simulink model "audioThru"  (R2020b)
settings: Solver=FixedStepDiscrete  StartTime=0.0  StopTime=10.0  RelTol=1e-3
settings Model: DataTypeOverride=Off  Creator=amatsumo  LastModifiedBy=amatsumo
settings DataIOCC: SaveOutput=off  SaveTime=off
settings OptimizationCC: BlockReduction=off  ConditionallyExecuteInputs=off  DefaultParameterBehavior=Inlined
settings DebuggingCC: AlgebraicLoopMsg=error  SingleTaskRateTransMsg=error  StrictBusMsg=ErrorOnBusTreatedAsVector  ArithmeticOperatorsInVariantConditions=warning
settings HardwareCC: ProdBitPerPointer=32  ProdBitPerSizeT=32  ProdBitPerPtrDiffT=32  ProdLargestAtomicFloat=None  ProdIntDivRoundTo=Undefined  ProdEndianess=Unspecified  ProdWordSize=32  ProdHWDeviceType=ASIC/FPGA->ASIC/FPGA  ProdEqTarget=off
settings SFSimCC: SimUseLocalCustomCode=off  CustomCodeUndefinedFunction=UseInterfaceOnly
settings RTWCC: RTWUseLocalCustomCode=off
settings CodeAppCC: StateflowObjectComments=on
settings GRTTargetCC: TargetLangStandard=C89/C90 (ANSI)

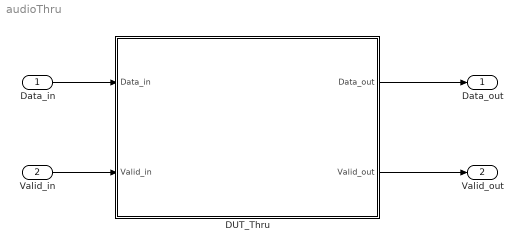
== system audioThru ==
  Data_in : Inport
  Valid_in : Inport  Port=2
  DUT_Thru : Subsystem  TreatAsAtomicUnit=on
  Data_out : Outport  VectorParamsAs1DForOutWhenUnconnected=off
  Valid_out : Outport  Port=2  VectorParamsAs1DForOutWhenUnconnected=off
  wires:
  DUT_Thru/1(Data_out) -> Data_out/1
  Data_in/1 -> DUT_Thru/1(Data_in)
  DUT_Thru/2(Valid_out) -> Valid_out/1
  Valid_in/1 -> DUT_Thru/2(Valid_in)

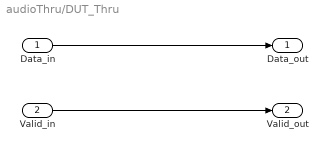
== system audioThru/DUT_Thru ==
  Data_in : Inport  OutDataTypeStr=fixdt(0,48,0)
  Valid_in : Inport  Port=2  OutDataTypeStr=boolean
  Data_out : Outport  OutDataTypeStr=fixdt(0,48,0)  VectorParamsAs1DForOutWhenUnconnected=off
  Valid_out : Outport  Port=2  OutDataTypeStr=boolean  VectorParamsAs1DForOutWhenUnconnected=off
  wires:
  Data_in/1 -> Data_out/1
  Valid_in/1 -> Valid_out/1
